simulink model "codegen_model"  (R2023b)
settings: Solver=FixedStepAuto  StartTime=0.0  StopTime=30  FixedStep=0.01  RelTol=1e-3
values from neighbouring files (symbols this model uses):
  abcs_deploy = 2000    [apogee_var.mat]    (also in step1_simtime_calculator_script.m)
  D = GlobalBest.Position(3)    [PSO_script.m]    (also in pid_var.mat = 92.8732132811)
  dy_mat = cell2mat(dy_mat_raw)    [step2_trajectories_sim_script.m]    (also in trajectories.mat = [7823.79537584 7362.53636793 6901.27736001 6440.01835209 597)
  I = GlobalBest.Position(2)    [PSO_script.m]    (also in pid_var.mat = 1)
  N = GlobalBest.Position(4)    [PSO_script.m]    (also in pid_var.mat = 138.62756105)
  P = GlobalBest.Position(1)    [PSO_script.m]    (also in pid_var.mat = 300)
  rate_lim = 1.85    [rocketdata.mat]    (also in step0_initialize_values.m)
  y = cell(1, 11)    [step2_trajectories_sim_script.m]    (also in trajectories.mat = )
libraries: simulink x1, slpidlib x1
settings Model: Creator=Alexinhow  LastModifiedBy=aless
settings OptimizationCC: DefaultParameterBehavior=Inlined  EnhancedBackFolding=on  PassReuseOutputArgsThreshold=0  OptimizeBlockOrder=speed  DifferentSizesBufferReuse=on  OptimizationCustomize=off
settings DebuggingCC: ParameterTunabilityLossMsg=error
settings SFSimCC: MATLABDynamicMemAlloc=off
settings RTWCC: Toolchain=MinGW64 | CMake/gmake (64-bit Windows)  BuildConfiguration=Release
settings CodeAppCC: ForceParamTrailComments=on  OperatorAnnotations=on

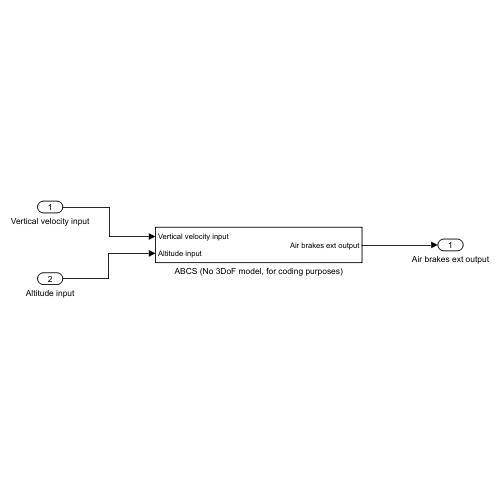
[thumbnail: Simulink's stored preview of the top-level diagram]
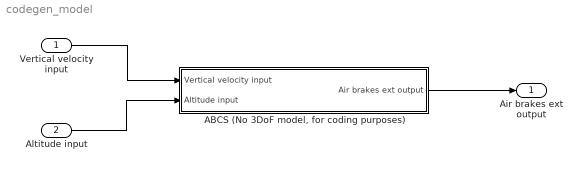
== system codegen_model ==
  Vertical velocity input : Inport
  Altitude input : Inport  Port=2
  "ABCS (No 3DoF model, for coding purposes)" : Subsystem
  Air brakes ext output : Outport
  wires:
  Vertical velocity input/1 -> "ABCS (No 3DoF model, for coding purposes)"/1(Vertical velocity input)
  Altitude input/1 -> "ABCS (No 3DoF model, for coding purposes)"/2(Altitude input)
  "ABCS (No 3DoF model, for coding purposes)"/1(Air brakes ext output) -> Air brakes ext output/1

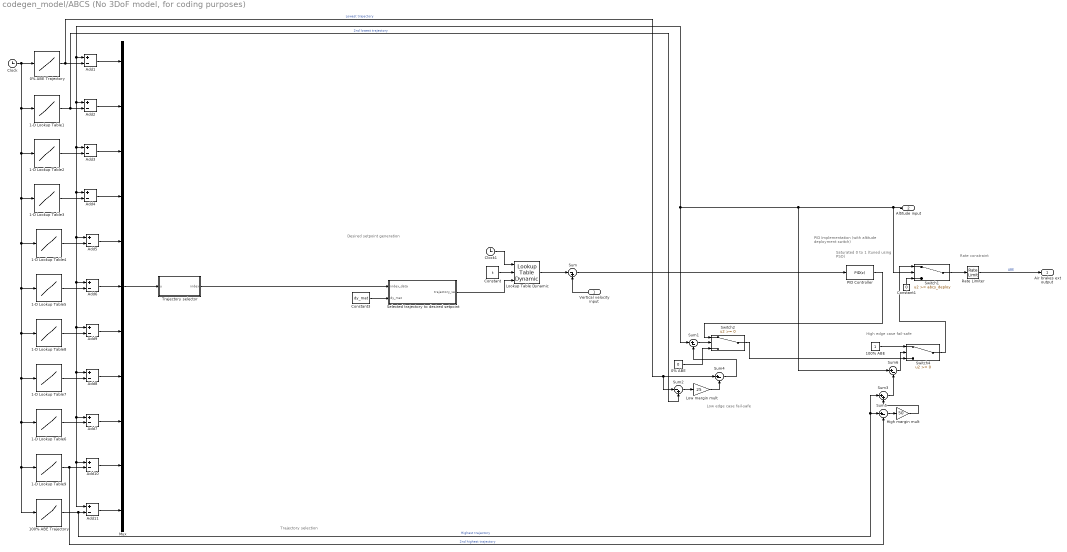
== system codegen_model/ABCS (No 3DoF model, for coding purposes) ==
  note: Rate constraint
  note: Saturated 0 to 1
      | (tuned using PSO)
  note: High edge case fail-safe
  note: Low edge case fail-safe
  note: Desired setpoint generation
  note: PID Implementation
      | (with altitude deployment switch)
  note: Trajectory selection
  Vertical velocity input : Inport
  Altitude input : Inport  Port=2
  0% ABE : Constant  Value=0
  0% ABE Trajectory : Lookup_n-D  NumberOfTableDimensions=1  BreakpointsForDimension1=y{1}.Time  Table=y{1}.Data  InternalRulePriority=Speed  RndMeth=Simplest
  1-D Lookup Table1 : Lookup_n-D  NumberOfTableDimensions=1  BreakpointsForDimension1=y{2}.Time  Table=y{2}.Data  InternalRulePriority=Speed  RndMeth=Simplest
  1-D Lookup Table2 : Lookup_n-D  NumberOfTableDimensions=1  BreakpointsForDimension1=y{3}.Time  Table=y{3}.Data  InternalRulePriority=Speed  RndMeth=Simplest
  1-D Lookup Table3 : Lookup_n-D  NumberOfTableDimensions=1  BreakpointsForDimension1=y{4}.Time  Table=y{4}.Data  InternalRulePriority=Speed  RndMeth=Simplest
  1-D Lookup Table4 : Lookup_n-D  NumberOfTableDimensions=1  BreakpointsForDimension1=y{5}.Time  Table=y{5}.Data  InternalRulePriority=Speed  RndMeth=Simplest
  1-D Lookup Table5 : Lookup_n-D  NumberOfTableDimensions=1  BreakpointsForDimension1=y{6}.Time  Table=y{6}.Data  InternalRulePriority=Speed  RndMeth=Simplest
  1-D Lookup Table6 : Lookup_n-D  NumberOfTableDimensions=1  BreakpointsForDimension1=y{9}.Time  Table=y{9}.Data  InternalRulePriority=Speed  RndMeth=Simplest
  1-D Lookup Table7 : Lookup_n-D  NumberOfTableDimensions=1  BreakpointsForDimension1=y{8}.Time  Table=y{8}.Data  InternalRulePriority=Speed  RndMeth=Simplest
  1-D Lookup Table8 : Lookup_n-D  NumberOfTableDimensions=1  BreakpointsForDimension1=y{7}.Time  Table=y{7}.Data  InternalRulePriority=Speed  RndMeth=Simplest
  1-D Lookup Table9 : Lookup_n-D  NumberOfTableDimensions=1  BreakpointsForDimension1=y{10}.Time  Table=y{10}.Data  InternalRulePriority=Speed  RndMeth=Simplest
  100% ABE : Constant
  100% ABE Trajectory : Lookup_n-D  NumberOfTableDimensions=1  BreakpointsForDimension1=y{11}.Time  Table=y{11}.Data  InternalRulePriority=Speed  RndMeth=Simplest
  Add{1..11} (11 alike) : Sum  Inputs=+-
  Clock : Clock
  Clock1 : Clock
  Constant : Constant  Value=t
  Constant1 : Constant  Value=0
  Constant3 : Constant  Value=dy_mat  SampleTime=0
  High margin mult : Gain  Gain=50
  Lookup Table Dynamic : simulink/Lookup Tables/Lookup Table Dynamic  LookUpMeth=Interpolation-Use End Values  OutDataType=fixdt('double')  OutScaling=[]  OutputDataTypeScalingMode=Specify via dialog  OutDataTypeStr=double  DoSatur=off
  Low margin mult : Gain  Gain=25
  Mux : Mux  Inputs=11
  PID Controller : slpidlib/PID Controller  Controller=PID  Form=Parallel  TimeDomain=Discrete-time  UseExternalTs=off  SampleTime=0.01  IntegratorMethod=Forward Euler  FilterMethod=Forward Euler  ControllerParametersSource=internal  P=P  I=I  UseKiTs=off  D=D  N=N  UseFilter=on  TunerSelectOption=Transfer Function Based (PID Tuner App)  InitialConditionSource=internal  InitialConditionForIntegrator=0  InitialConditionForFilter=0  DifferentiatorICPrevScaledInput=0  ExternalReset=none  TrackingMode=off  Kt=1  LimitOutput=on  SatLimitsSource=internal  UpperSaturationLimit=1  LowerSaturationLimit=0  LinearizeAsGain=off  AntiWindupMode=none  Kb=1  LimitIntegrator=off  UpperIntegratorSaturationLimit=inf  LowerIntegratorSaturationLimit=-inf  POutMin=[]  POutMax=[]  IOutMin=[]  IOutMax=[]  DOutMin=[]  DOutMax=[]  NOutMin=[]  NOutMax=[]  SumOutMin=[]  SumOutMax=[]  SaturationOutMin=[]  SaturationOutMax=[]  PParamMin=[]  PParamMax=[]  IParamMin=[]  IParamMax=[]  DParamMin=[]  DParamMax=[]  NParamMin=[]  NParamMax=[]  KbParamMin=[]  KbParamMax=[]  KtParamMin=[]  KtParamMax=[]  KbOutMin=[]  KbOutMax=[]  KtOutMin=[]  KtOutMax=[]  IntegratorOutMin=[]  IntegratorOutMax=[]  FilterOutMin=[]  FilterOutMax=[]  SumI1OutMin=[]  SumI1OutMax=[]  SumI2OutMin=[]  SumI2OutMax=[]  SumI3OutMin=[]  SumI3OutMax=[]  SumI4OutMin=[]  SumI4OutMax=[]  SumDOutMin=[]  SumDOutMax=[]  DifferentiatorOutMin=[]  DifferentiatorOutMax=[]  FilterDiffOutCoefMin=[]  FilterDiffOutCoefMax=[]  ReciprocalOutMin=[]  ReciprocalOutMax=[]  SumDenOutMin=[]  SumDenOutMax=[]  SumNumOutMin=[]  SumNumOutMax=[]  DivideOutMin=[]  DivideOutMax=[]  UdiffTsProdOutMin=[]  UdiffTsProdOutMax=[]  NTsProdOutMin=[]  NTsProdOutMax=[]  UintegralTsProdOutMin=[]  UintegralTsProdOutMax=[]  UngainTsProdOutMin=[]  UngainTsProdOutMax=[]  ClampingZeroOutDataTypeStr=Inherit: Inherit via back propagation  ClampingZeroOutMin=[]  ClampingZeroOutMax=[]  FilterDenConstantOutDataTypeStr=Inherit: Inherit via back propagation  FilterDenConstantOutMin=[]  FilterDenConstantOutMax=[]  PCopyOutDataTypeStr=Inherit: Inherit via back propagation  PCopyOutMin=[]  PCopyOutMax=[]  NCopyOutDataTypeStr=Inherit: Inherit via back propagation  NCopyOutMin=[]  NCopyOutMax=[]  IntegratorContinuousStateAttributes=''  IntegratorStateMustResolveToSignalObject=off  IntegratorRTWStateStorageClass=Auto  FilterContinuousStateAttributes=''  FilterStateMustResolveToSignalObject=off  FilterRTWStateStorageClass=Auto  ParallelPVariant=InternalParameters  IdealPVariant=Disabled  IVariant=InternalParameters  DVariant=InternalParameters  IntegratorVariant=Discrete  SatVariant=Enabled  AWVariant=Passthrough  PCopyVariant=Disabled  TRVariant=Disabled  FdbkBlocksVariant=Forward  IdealPFdbkVariant=Disabled  SatFdbkVariant=Disabled  DerivativeFilterVariant=ForwardEulerFilter  NVariant=InternalParameters  NCopyVariant=Disabled  FilterICVariant=InternalICsFilter  IntegratorICVariant=InternalICs  ExternalResetVariant=Disabled  TRSumVariant=Passthrough  SumFdbkVariant=Disabled  SumVariant=Sum_PID  TsampFilterVariant=InternalTs  TsampNgainVariant=Passthrough  TsampIntegralVariant=Disabled_SignalSpec  ExternalSaturationOutDataTypeStr=Inherit: Same as second input
  Rate Limiter : RateLimiter  RisingSlewLimit=rate_lim  FallingSlewLimit=-rate_lim  SampleTimeMode=inherited
  Selected trajectory to desired setpoint : MATLAB Function  TreatAsAtomicUnit=on
  Sum : Sum  Inputs=|-+
  Sum{1,4..6} (4 alike) : Sum  Inputs=|+-
  Sum2 : Sum  Inputs=|-+
  Sum3 : Sum  Inputs=|++
  Switch1 : Switch  Threshold=abcs_deploy  SaturateOnIntegerOverflow=off  InputSameDT=off
  Switch2 : Switch  SaturateOnIntegerOverflow=off  InputSameDT=off
  Switch4 : Switch  SaturateOnIntegerOverflow=off  InputSameDT=off
  Trajectory selector : MATLAB Function  TreatAsAtomicUnit=on
  Air brakes ext output : Outport
  wires:
  Mux/1 -> Trajectory selector/1(u)
  1-D Lookup Table4/1 -> Add5/2
  Switch2/1 -> Switch4/3
  Sum1/1 -> Switch2/2
  Altitude input/1 -> Switch1/2, Add3/1, Add4/1, Add5/1, Add6/1, Add9/1, Add8/1, Add7/1, Add10/1, Add11/1, Add2/1, Add1/1, Sum1/1, Sum6/1
  Clock/1 -> 1-D Lookup Table5/1, 1-D Lookup Table8/1, 1-D Lookup Table7/1, 1-D Lookup Table6/1, 1-D Lookup Table9/1, 100% ABE Trajectory/1, 1-D Lookup Table4/1, 1-D Lookup Table3/1, 1-D Lookup Table2/1, 1-D Lookup Table1/1, 0% ABE Trajectory/1
  1-D Lookup Table5/1 -> Add6/2
  Lookup Table Dynamic/1 -> Sum/1
  Rate Limiter/1 -> Air brakes ext output/1  "ABE"
  1-D Lookup Table1/1 -> Add2/2, Sum2/2  "2nd lowest trajectory"
  Vertical velocity input/1 -> Sum/2
  Add6/1 -> Mux/6
  Sum/1 -> PID Controller/1
  Add11/1 -> Mux/11
  Add10/1 -> Mux/10
  Trajectory selector/1(index) -> Selected trajectory to desired setpoint/1(index_data)
  Add4/1 -> Mux/4
  1-D Lookup Table9/1 -> Sum5/2, Add10/2  "2nd highest trajectory"
  0% ABE Trajectory/1 -> Add1/2, Sum2/1, Sum4/1  "Lowest trajectory"
  1-D Lookup Table6/1 -> Add7/2
  Add2/1 -> Mux/2
  100% ABE Trajectory/1 -> Add11/2, Sum3/1, Sum5/1  "Highest trajectory"
  Constant/1 -> Lookup Table Dynamic/2
  Add3/1 -> Mux/3
  Add5/1 -> Mux/5
  Add7/1 -> Mux/9
  PID Controller/1 -> Switch2/1
  Add8/1 -> Mux/8
  1-D Lookup Table8/1 -> Add9/2
  Sum3/1 -> Sum6/2
  Constant3/1 -> Selected trajectory to desired setpoint/2(dy_mat)
  High margin mult/1 -> Sum3/2
  Add1/1 -> Mux/1
  Sum4/1 -> Sum1/2
  1-D Lookup Table3/1 -> Add4/2
  Sum2/1 -> Low margin mult/1
  Clock1/1 -> Lookup Table Dynamic/1
  Low margin mult/1 -> Sum4/2
  Add9/1 -> Mux/7
  Selected trajectory to desired setpoint/1(trajectory_vel) -> Lookup Table Dynamic/3
  Sum6/1 -> Switch4/2
  Sum5/1 -> High margin mult/1
  1-D Lookup Table2/1 -> Add3/2
  1-D Lookup Table7/1 -> Add8/2
  Constant1/1 -> Switch1/3
  0% ABE/1 -> Switch2/3
  100% ABE/1 -> Switch4/1
  Switch1/1 -> Rate Limiter/1
  Switch4/1 -> Switch1/1

== matlab function codegen_model/ABCS (No 3DoF model, for coding purposes)/Selected trajectory to desired setpoint ==
  data: index_data input; trajectory_vel output; dy_mat input
function trajectory_vel = index2traj_vel(index_data,dy_mat)
trajectory_vel = dy_mat(:,index_data);

== matlab function codegen_model/ABCS (No 3DoF model, for coding purposes)/Trajectory selector ==
  data: u input; index output
function index = traj_selector(u)
    
    min_difference = Inf;
    index_of_closest = 0;

    
    for i = 1:length(u)
        
        difference = abs(u(i) - 0);
        
        if difference < min_difference
            
            min_difference = difference;
            index_of_closest = i;
        end
    end
    
    index = index_of_closest;
end
